simulink model "AIN_3x_6VT"  (R2018b)
settings: Solver=ode23t  StartTime=0.0  StopTime=0.3  RelTol=1e-3
undefined symbols (not defined in the file): C, DiscIntNeverNeededParam, fout, L, Rn
libraries: powerlib x38, powerlib_meascontrol x5, peRmsMeasurement x2, dspstat3 x1
settings Model: Creator=K2  LastModifiedBy=VID Company

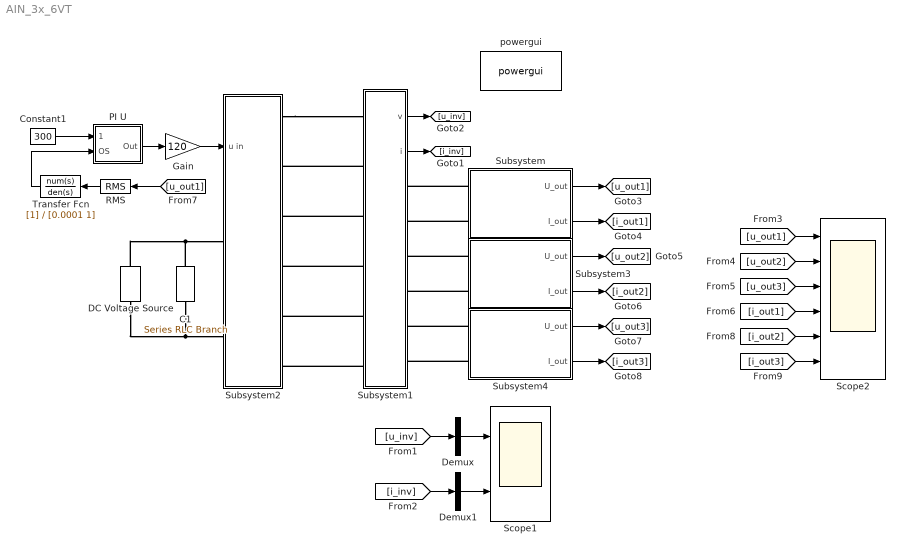
== system AIN_3x_6VT ==
  C1 : powerlib/Elements/Series RLC Branch  LConnTagsString=__new0  RConnTagsString=__new0  BranchType=RC  Resistance=0.050  Inductance=1e-3  SetiL0=off  InitialCurrent=0  Capacitance=10000e-6  Setx0=off  InitialVoltage=0  Measurements=None
  Constant1 : Constant  Value=300  SampleTime=1e-6
  DC Voltage Source : powerlib/Electrical Sources/DC Voltage Source  Amplitude=500  Measurements=None
  Demux : Demux  Outputs=3
  Demux1 : Demux  Outputs=3
  Gain : Gain  Gain=120
  PI U : Subsystem
  RMS : powerlib_meascontrol/Measurements/RMS  TrueRMS=off  Freq=400  RMSInit=0  Ts=0
  Scope1 : Scope  NumInputPorts=2
  Scope2 : Scope  NumInputPorts=6
  Subsystem : Subsystem
  Subsystem1 : Subsystem
  Subsystem2 : Subsystem
  Subsystem3 : Subsystem
  Subsystem4 : Subsystem
  Transfer Fcn : TransferFcn  Denominator=[0.0001 1]
  powergui : powerlib/powergui  Priority=1  SimulationMode=Discrete  SampleTime=1e-7  frequency=60  Iterations=50  frequencyindice=0  Pbase=100e6  ErrMax=1e-4  UnitsV=kV  UnitsW=MW  buscounter=0  FunctionMessages=off  echomessages=off  EnableUseOfTLC=off  CurrentSourceSwitches=off  DisableSnubberDevices=off  DisableRonSwitches=off  DisableVfSwitches=off  DisplayEquations=off  SolverType=Tustin/Backward Euler (TBE)  Interpol=off  ExternalGateDelay=off  methode=off  Ts=100  x0status=blocks  SPID=on  SwTol=0  HookPort=off  RestoreLinks=warning  ResistiveCurrentMeasurement=off  Frange=[0:2:500]  Ylog=off  Xlog=on  ShowGrid=off  save=off  variable=ZData  structure=logsout  ZoomFFT=on  StartTime=0.28  cycles=4  DisplayStyle=1  fundamental=400  FreqAxis=off  MaxFrequency=20000  frequencyindicesteady=1  RmsSteady=1  display=off
  wires:
  Constant1/1 -> PI U/1(Zad)
  RMS/1 -> Transfer Fcn/1
  Gain/1 -> Subsystem2/1(u in)
  PI U/1(Out) -> Gain/1
  Transfer Fcn/1 -> PI U/2(OS)
  Subsystem1/2(i) -> [i_inv]
  Subsystem1/1(v) -> [u_inv]
  [u_out1] -> RMS/1
  Subsystem/1(U_out) -> [u_out1]
  Subsystem/2(I_out) -> [i_out1]
  Subsystem3/1(U_out) -> [u_out2]
  Subsystem3/2(I_out) -> [i_out2]
  Subsystem4/1(U_out) -> [u_out3]
  Subsystem4/2(I_out) -> [i_out3]
  [u_out1] -> Scope2/1
  [u_out2] -> Scope2/2
  [u_out3] -> Scope2/3
  [i_out1] -> Scope2/4
  [i_out2] -> Scope2/5
  [i_out3] -> Scope2/6
  [u_inv] -> Demux/1
  [i_inv] -> Demux1/1
  Demux/2 -> Scope1/1
  Demux1/2 -> Scope1/2
  connections:
  DC Voltage Source/RConn1 -- C1/LConn1 -- Subsystem2/LConn1
  DC Voltage Source/LConn1 -- C1/RConn1 -- Subsystem2/LConn2
  Subsystem2/RConn1 -- Subsystem1/LConn1
  Subsystem1/LConn2 -- Subsystem2/RConn2
  Subsystem1/LConn4 -- Subsystem2/RConn4
  Subsystem1/LConn3 -- Subsystem2/RConn3
  Subsystem1/LConn5 -- Subsystem2/RConn5
  Subsystem1/LConn6 -- Subsystem2/RConn6
  Subsystem/LConn1 -- Subsystem1/RConn1
  Subsystem/LConn2 -- Subsystem1/RConn2
  Subsystem3/LConn1 -- Subsystem1/RConn3
  Subsystem3/LConn2 -- Subsystem1/RConn4
  Subsystem4/LConn1 -- Subsystem1/RConn5
  Subsystem4/LConn2 -- Subsystem1/RConn6

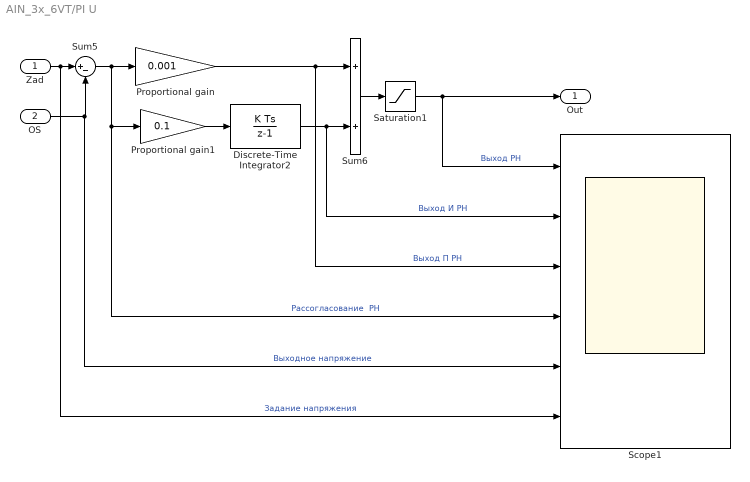
== system AIN_3x_6VT/PI U ==
  Zad : Inport
  OS : Inport  Port=2
  Discrete-Time Integrator2 : DiscreteIntegrator  SampleTime=-1  LimitOutput=on  UpperSaturationLimit=1  LowerSaturationLimit=0  ICPrevOutput=DiscIntNeverNeededParam  ICPrevScaledInput=DiscIntNeverNeededParam
  Proportional gain : Gain  Gain=0.001  SaturateOnIntegerOverflow=on  OutDataTypeStr=Inherit: Same as input  ParamDataTypeStr=Inherit: Same as input
  Proportional gain1 : Gain  Gain=0.1  SaturateOnIntegerOverflow=on  OutDataTypeStr=Inherit: Same as input  ParamDataTypeStr=Inherit: Same as input
  Saturation1 : Saturate  UpperLimit=1  LowerLimit=0
  Scope1 : Scope  NumInputPorts=6
  Sum5 : Sum  Inputs=|+-  SaturateOnIntegerOverflow=on  InputSameDT=on  OutDataTypeStr=Inherit: Same as first input
  Sum6 : Sum  SaturateOnIntegerOverflow=on  InputSameDT=on  OutDataTypeStr=Inherit: Same as first input
  Out : Outport
  wires:
  Proportional gain/1 -> Scope1/3, Sum6/1  "Выход П РН"
  Discrete-Time Integrator2/1 -> Sum6/2, Scope1/2  "Выход И РН"
  OS/1 -> Scope1/5, Sum5/2  "Выходное напряжение"
  Zad/1 -> Scope1/6, Sum5/1  "Задание напряжения"
  Sum5/1 -> Proportional gain1/1, Scope1/4, Proportional gain/1  "Рассогласование  РН"
  Sum6/1 -> Saturation1/1
  Saturation1/1 -> Out/1, Scope1/1  "Выход РН"
  Proportional gain1/1 -> Discrete-Time Integrator2/1

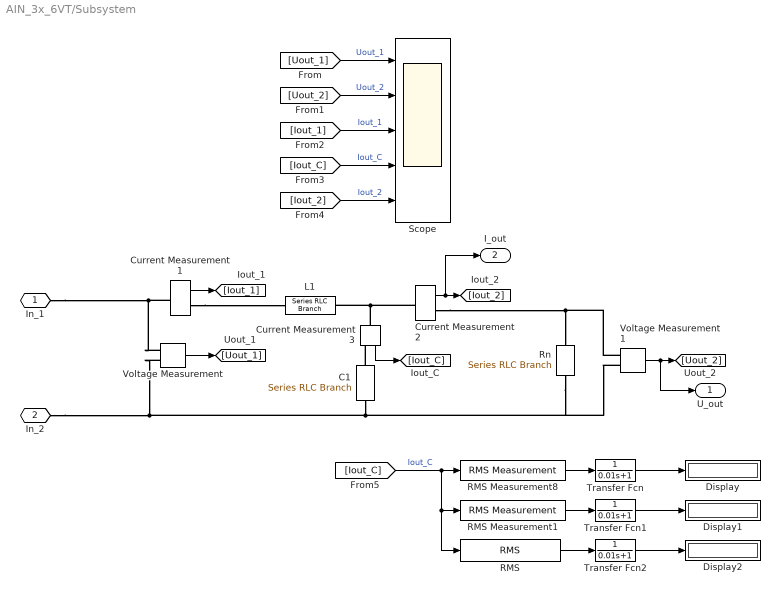
== system AIN_3x_6VT/Subsystem ==
  C1 : powerlib/Elements/Series RLC Branch  LConnTagsString=__new0  RConnTagsString=__new0  BranchType=RC  Resistance=0.050  Inductance=1e-3  SetiL0=off  InitialCurrent=0  Capacitance=C  Setx0=off  InitialVoltage=0  Measurements=None
  Current Measurement1 : powerlib/Measurements/Current Measurement  PhasorSimulation=off  OutputType=Complex  PSBequivalent=0
  Current Measurement2 : powerlib/Measurements/Current Measurement  PhasorSimulation=off  OutputType=Complex  PSBequivalent=0
  Current Measurement3 : powerlib/Measurements/Current Measurement  PhasorSimulation=off  OutputType=Complex  PSBequivalent=0
  Display : Display
  Display1 : Display
  Display2 : Display
  L1 : powerlib/Elements/Series RLC Branch  LConnTagsString=__new0  RConnTagsString=__new0  BranchType=RL  Resistance=0.1  Inductance=L  SetiL0=off  InitialCurrent=0  Capacitance=10e-3  Setx0=off  InitialVoltage=0  Measurements=None
  RMS : dspstat3/RMS  run=off  directionMode=Each column  dimension=1  InputProcessing=Columns as channels (frame based)  reset_popup=None
  RMS Measurement1 : peRmsMeasurement/RMS Measurement  LabelModeActiveChoice=Harmonic  F=8000  SpecifyHarmonics=on  K=[1]  Ts=0
  RMS Measurement8 : peRmsMeasurement/RMS Measurement  LabelModeActiveChoice=Harmonic  F=400  SpecifyHarmonics=on  K=[1]  Ts=0
  Rn : powerlib/Elements/Series RLC Branch  LConnTagsString=__new0  RConnTagsString=__new0  BranchType=RL  Resistance=Rn  Inductance=0.01e-3  SetiL0=off  InitialCurrent=0  Capacitance=50e-6  Setx0=off  InitialVoltage=0  Measurements=None
  Scope : Scope  NumInputPorts=5
  Transfer Fcn : TransferFcn  Denominator=[0.01 1]
  Transfer Fcn1 : TransferFcn  Denominator=[0.01 1]
  Transfer Fcn2 : TransferFcn  Denominator=[0.01 1]
  Voltage Measurement : powerlib/Measurements/Voltage Measurement  PhasorSimulation=off  OutputType=Complex  PSBequivalent=0
  Voltage Measurement1 : powerlib/Measurements/Voltage Measurement  PhasorSimulation=off  OutputType=Complex  PSBequivalent=0
  In_1 : PMIOPort  Side=Left
  In_2 : PMIOPort  Port=2  Side=Left
  U_out : Outport
  I_out : Outport  Port=2
  wires:
  Voltage Measurement1/1 -> U_out/1, [Uout_2]
  Current Measurement1/1 -> [Iout_1]
  Current Measurement2/1 -> I_out/1, [Iout_2]
  Voltage Measurement/1 -> [Uout_1]
  Current Measurement3/1 -> [Iout_C]
  [Iout_C] -> Scope/4  "Iout_C"
  [Uout_2] -> Scope/2  "Uout_2"
  [Iout_1] -> Scope/3  "Iout_1"
  [Iout_2] -> Scope/5  "Iout_2"
  [Uout_1] -> Scope/1  "Uout_1"
  [Iout_C] -> RMS/1, RMS Measurement1/1, RMS Measurement8/1  "Iout_C"
  RMS Measurement8/1 -> Transfer Fcn/1
  RMS Measurement1/1 -> Transfer Fcn1/1
  Transfer Fcn/1 -> Display/1
  Transfer Fcn1/1 -> Display1/1
  Transfer Fcn2/1 -> Display2/1
  RMS/1 -> Transfer Fcn2/1
  connections:
  Current Measurement3/LConn1 -- Current Measurement2/LConn1 -- L1/RConn1
  Current Measurement1/LConn1 -- In_1/RConn1 -- Voltage Measurement/LConn1
  Voltage Measurement/LConn2 -- In_2/RConn1 -- C1/RConn1 -- Rn/RConn1 -- Voltage Measurement1/LConn2
  Voltage Measurement1/LConn1 -- Current Measurement2/RConn1 -- Rn/LConn1
  Current Measurement1/RConn1 -- L1/LConn1
  C1/LConn1 -- Current Measurement3/RConn1

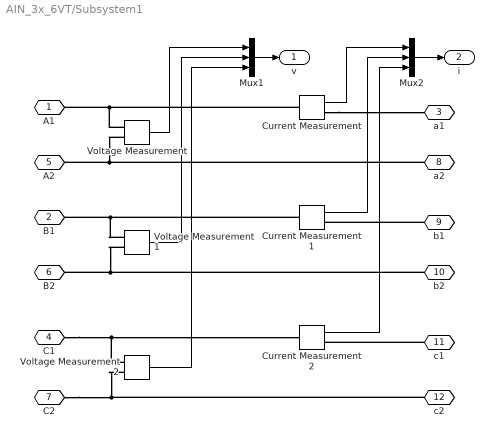
== system AIN_3x_6VT/Subsystem1 ==
  Current Measurement : powerlib/Measurements/Current Measurement  PhasorSimulation=off  OutputType=Complex  PSBequivalent=0
  Current Measurement1 : powerlib/Measurements/Current Measurement  PhasorSimulation=off  OutputType=Complex  PSBequivalent=0
  Current Measurement2 : powerlib/Measurements/Current Measurement  PhasorSimulation=off  OutputType=Complex  PSBequivalent=0
  Mux1 : Mux  Inputs=3
  Mux2 : Mux  Inputs=3
  Voltage Measurement : powerlib/Measurements/Voltage Measurement  PhasorSimulation=off  OutputType=Complex  PSBequivalent=0
  Voltage Measurement1 : powerlib/Measurements/Voltage Measurement  PhasorSimulation=off  OutputType=Complex  PSBequivalent=0
  Voltage Measurement2 : powerlib/Measurements/Voltage Measurement  PhasorSimulation=off  OutputType=Complex  PSBequivalent=0
  A1 : PMIOPort  Side=Left
  B1 : PMIOPort  Port=2  Side=Left
  a1 : PMIOPort  Port=3  Side=Right
  C1 : PMIOPort  Port=4  Side=Left
  A2 : PMIOPort  Port=5  Side=Left
  B2 : PMIOPort  Port=6  Side=Left
  C2 : PMIOPort  Port=7  Side=Left
  a2 : PMIOPort  Port=8  Side=Right
  b1 : PMIOPort  Port=9  Side=Right
  b2 : PMIOPort  Port=10  Side=Right
  c1 : PMIOPort  Port=11  Side=Right
  c2 : PMIOPort  Port=12  Side=Right
  v : Outport
  i : Outport  Port=2
  wires:
  Voltage Measurement1/1 -> Mux1/2
  Current Measurement2/1 -> Mux2/3
  Voltage Measurement2/1 -> Mux1/3
  Current Measurement/1 -> Mux2/1
  Voltage Measurement/1 -> Mux1/1
  Mux1/1 -> v/1
  Current Measurement1/1 -> Mux2/2
  Mux2/1 -> i/1
  connections:
  Current Measurement/RConn1 -- a1/RConn1
  Current Measurement/LConn1 -- Voltage Measurement/LConn1 -- A1/RConn1
  C1/RConn1 -- Voltage Measurement2/LConn1 -- Current Measurement2/LConn1
  c1/RConn1 -- Current Measurement2/RConn1
  Current Measurement1/LConn1 -- Voltage Measurement1/LConn1 -- B1/RConn1
  b1/RConn1 -- Current Measurement1/RConn1
  Voltage Measurement/LConn2 -- a2/RConn1 -- A2/RConn1
  Voltage Measurement1/LConn2 -- b2/RConn1 -- B2/RConn1
  Voltage Measurement2/LConn2 -- c2/RConn1 -- C2/RConn1

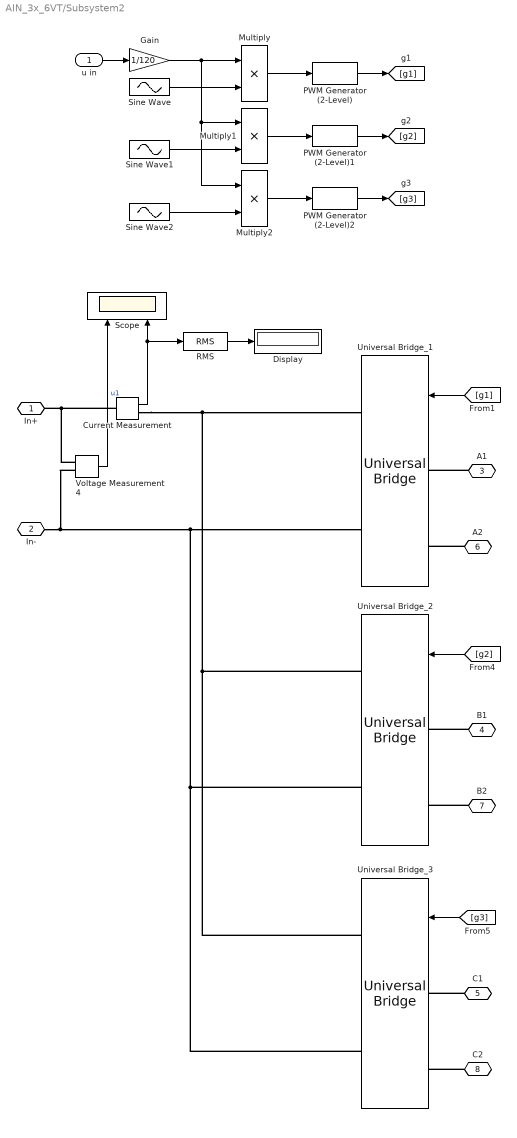
== system AIN_3x_6VT/Subsystem2 ==
  u in : Inport
  Current Measurement : powerlib/Measurements/Current Measurement  PhasorSimulation=off  OutputType=Complex  PSBequivalent=0
  Display : Display
  Gain : Gain  Gain=1/120
  Multiply : Product
  Multiply1 : Product
  Multiply2 : Product
  PWM Generator (2-Level) : powerlib_meascontrol/Pulse & Signal Generators/PWM Generator (2-Level)  ModulatorType=Single-phase full-bridge (4 pulses)  ModulatorMode=Unsynchronized  Fc=fPWM  Pc=0  nF=27  MinMax="[ -1  1 ]"  SamplingTechnique=Symmetrical regular (single edge)  ModulatingSignals=off  m=0.8  Freq=60  Phase=0  Ts=0  ShowCarrierOutport=off
      settings: SourceProductName=Simscape Power Systems
  PWM Generator (2-Level)1 : powerlib_meascontrol/Pulse & Signal Generators/PWM Generator (2-Level)  ModulatorType=Single-phase full-bridge (4 pulses)  ModulatorMode=Unsynchronized  Fc=fPWM  Pc=120  nF=27  MinMax="[ -1  1 ]"  SamplingTechnique=Symmetrical regular (single edge)  ModulatingSignals=off  m=0.8  Freq=60  Phase=0  Ts=0  ShowCarrierOutport=off
      settings: SourceProductName=Simscape Power Systems
  PWM Generator (2-Level)2 : powerlib_meascontrol/Pulse & Signal Generators/PWM Generator (2-Level)  ModulatorType=Single-phase full-bridge (4 pulses)  ModulatorMode=Unsynchronized  Fc=fPWM  Pc=240  nF=27  MinMax="[ -1  1 ]"  SamplingTechnique=Symmetrical regular (single edge)  ModulatingSignals=off  m=0.8  Freq=60  Phase=0  Ts=0  ShowCarrierOutport=off
      settings: SourceProductName=Simscape Power Systems
  RMS : powerlib_meascontrol/Measurements/RMS  TrueRMS=on  Freq=60  RMSInit=120  Ts=0
  Scope : Scope  NumInputPorts=2
  Sine Wave : Sin  Amplitude=0.99  Frequency=fout*2*pi  SampleTime=0
  Sine Wave1 : Sin  Amplitude=0.99  Frequency=fout*2*pi  Phase=2*pi*fout*(120/360)  SampleTime=0
  Sine Wave2 : Sin  Amplitude=0.99  Frequency=fout*2*pi  Phase=2*pi*fout*(240/360)  SampleTime=0
  Universal Bridge_1 : powerlib/Power Electronics/Universal Bridge  Arms=2  SnubberResistance=1e5  SnubberCapacitance=inf  Device=IGBT / Diodes  Ron=5e-3  Lon=0  ForwardVoltages="[  1.5  1  ]"  ForwardVoltage=0  GTOparameters=[ 10e-6 , 20e-6 ]  IGBTparameters=[ 1e-6 , 2e-6 ]  Measurements=Device currents  Measurements_2=None  converterType=Rectifier
  Universal Bridge_2 : powerlib/Power Electronics/Universal Bridge  Arms=2  SnubberResistance=1e5  SnubberCapacitance=inf  Device=IGBT / Diodes  Ron=5e-3  Lon=0  ForwardVoltages="[  1.5  1  ]"  ForwardVoltage=0  GTOparameters=[ 10e-6 , 20e-6 ]  IGBTparameters=[ 1e-6 , 2e-6 ]  Measurements=None  Measurements_2=None  converterType=Rectifier
  Universal Bridge_3 : powerlib/Power Electronics/Universal Bridge  Arms=2  SnubberResistance=1e5  SnubberCapacitance=inf  Device=IGBT / Diodes  Ron=5e-3  Lon=0  ForwardVoltages="[  1.5  1  ]"  ForwardVoltage=0  GTOparameters=[ 10e-6 , 20e-6 ]  IGBTparameters=[ 1e-6 , 2e-6 ]  Measurements=None  Measurements_2=None  converterType=Rectifier
  Voltage Measurement4 : powerlib/Measurements/Voltage Measurement  PhasorSimulation=off  OutputType=Complex  PSBequivalent=0
  In+ : PMIOPort  Side=Left
  In- : PMIOPort  Port=2  Side=Left
  A1 : PMIOPort  Port=3  Side=Right
  B1 : PMIOPort  Port=4  Side=Right
  C1 : PMIOPort  Port=5  Side=Right
  A2 : PMIOPort  Port=6  Side=Right
  B2 : PMIOPort  Port=7  Side=Right
  C2 : PMIOPort  Port=8  Side=Right
  wires:
  PWM Generator (2-Level)/1 -> [g1]
  Gain/1 -> Multiply2/1, Multiply1/1, Multiply/1
  u in/1 -> Gain/1
  Multiply/1 -> PWM Generator (2-Level)/1
  Sine Wave/1 -> Multiply/2
  Current Measurement/1 -> RMS/1, Scope/2
  Voltage Measurement4/1 -> Scope/1  "u1"
  Multiply1/1 -> PWM Generator (2-Level)1/1
  Multiply2/1 -> PWM Generator (2-Level)2/1
  PWM Generator (2-Level)2/1 -> [g3]
  PWM Generator (2-Level)1/1 -> [g2]
  [g1] -> Universal Bridge_1/1
  [g2] -> Universal Bridge_2/1
  [g3] -> Universal Bridge_3/1
  Sine Wave2/1 -> Multiply2/2
  Sine Wave1/1 -> Multiply1/2
  RMS/1 -> Display/1
  connections:
  Current Measurement/LConn1 -- Voltage Measurement4/LConn1 -- In+/RConn1
  In-/RConn1 -- Voltage Measurement4/LConn2 -- Universal Bridge_3/RConn2 -- Universal Bridge_2/RConn2 -- Universal Bridge_1/RConn2
  Current Measurement/RConn1 -- Universal Bridge_2/RConn1 -- Universal Bridge_3/RConn1 -- Universal Bridge_1/RConn1
  A1/RConn1 -- Universal Bridge_1/LConn1
  B1/RConn1 -- Universal Bridge_2/LConn1
  C1/RConn1 -- Universal Bridge_3/LConn1
  A2/RConn1 -- Universal Bridge_1/LConn2
  B2/RConn1 -- Universal Bridge_2/LConn2
  C2/RConn1 -- Universal Bridge_3/LConn2

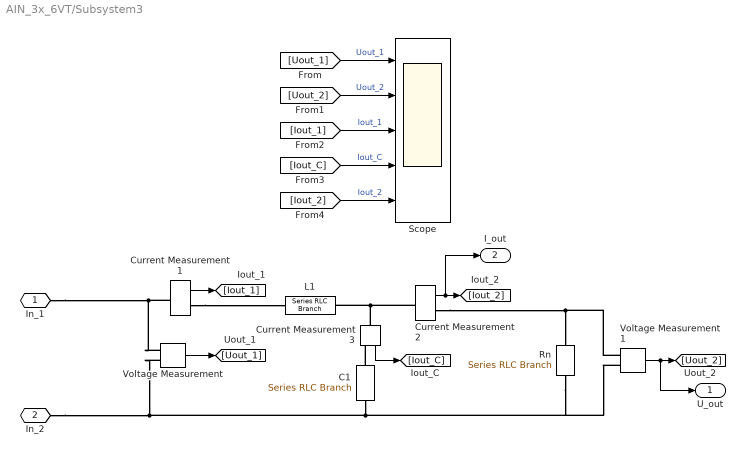
== system AIN_3x_6VT/Subsystem3 ==
  C1 : powerlib/Elements/Series RLC Branch  LConnTagsString=__new0  RConnTagsString=__new0  BranchType=RC  Resistance=0.050  Inductance=1e-3  SetiL0=off  InitialCurrent=0  Capacitance=C  Setx0=off  InitialVoltage=0  Measurements=None
  Current Measurement1 : powerlib/Measurements/Current Measurement  PhasorSimulation=off  OutputType=Complex  PSBequivalent=0
  Current Measurement2 : powerlib/Measurements/Current Measurement  PhasorSimulation=off  OutputType=Complex  PSBequivalent=0
  Current Measurement3 : powerlib/Measurements/Current Measurement  PhasorSimulation=off  OutputType=Complex  PSBequivalent=0
  L1 : powerlib/Elements/Series RLC Branch  LConnTagsString=__new0  RConnTagsString=__new0  BranchType=RL  Resistance=0.1  Inductance=L  SetiL0=off  InitialCurrent=0  Capacitance=10e-3  Setx0=off  InitialVoltage=0  Measurements=None
  Rn : powerlib/Elements/Series RLC Branch  LConnTagsString=__new0  RConnTagsString=__new0  BranchType=RL  Resistance=Rn  Inductance=0.01e-3  SetiL0=off  InitialCurrent=0  Capacitance=50e-6  Setx0=off  InitialVoltage=0  Measurements=None
  Scope : Scope  NumInputPorts=5
  Voltage Measurement : powerlib/Measurements/Voltage Measurement  PhasorSimulation=off  OutputType=Complex  PSBequivalent=0
  Voltage Measurement1 : powerlib/Measurements/Voltage Measurement  PhasorSimulation=off  OutputType=Complex  PSBequivalent=0
  In_1 : PMIOPort  Side=Left
  In_2 : PMIOPort  Port=2  Side=Left
  U_out : Outport
  I_out : Outport  Port=2
  wires:
  Voltage Measurement1/1 -> U_out/1, [Uout_2]
  Current Measurement1/1 -> [Iout_1]
  Current Measurement2/1 -> I_out/1, [Iout_2]
  Voltage Measurement/1 -> [Uout_1]
  Current Measurement3/1 -> [Iout_C]
  [Iout_C] -> Scope/4  "Iout_C"
  [Uout_2] -> Scope/2  "Uout_2"
  [Iout_1] -> Scope/3  "Iout_1"
  [Iout_2] -> Scope/5  "Iout_2"
  [Uout_1] -> Scope/1  "Uout_1"
  connections:
  Current Measurement3/LConn1 -- Current Measurement2/LConn1 -- L1/RConn1
  Current Measurement1/LConn1 -- In_1/RConn1 -- Voltage Measurement/LConn1
  Voltage Measurement/LConn2 -- In_2/RConn1 -- C1/RConn1 -- Rn/RConn1 -- Voltage Measurement1/LConn2
  Voltage Measurement1/LConn1 -- Current Measurement2/RConn1 -- Rn/LConn1
  Current Measurement1/RConn1 -- L1/LConn1
  C1/LConn1 -- Current Measurement3/RConn1

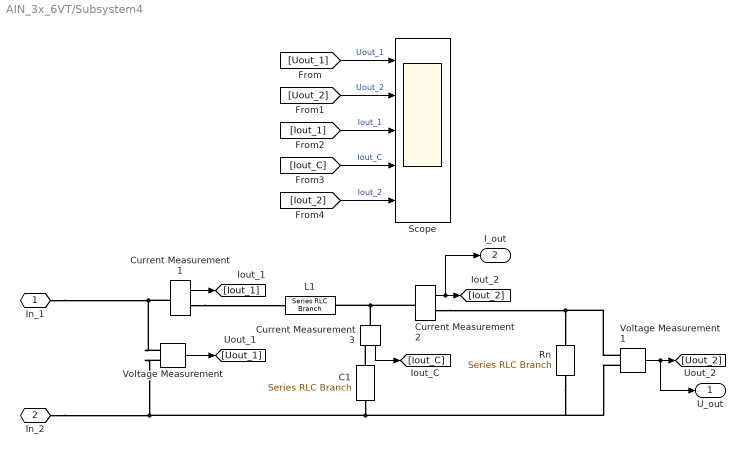
== system AIN_3x_6VT/Subsystem4 ==
  C1 : powerlib/Elements/Series RLC Branch  LConnTagsString=__new0  RConnTagsString=__new0  BranchType=RC  Resistance=0.050  Inductance=1e-3  SetiL0=off  InitialCurrent=0  Capacitance=C  Setx0=off  InitialVoltage=0  Measurements=None
  Current Measurement1 : powerlib/Measurements/Current Measurement  PhasorSimulation=off  OutputType=Complex  PSBequivalent=0
  Current Measurement2 : powerlib/Measurements/Current Measurement  PhasorSimulation=off  OutputType=Complex  PSBequivalent=0
  Current Measurement3 : powerlib/Measurements/Current Measurement  PhasorSimulation=off  OutputType=Complex  PSBequivalent=0
  L1 : powerlib/Elements/Series RLC Branch  LConnTagsString=__new0  RConnTagsString=__new0  BranchType=RL  Resistance=0.1  Inductance=L  SetiL0=off  InitialCurrent=0  Capacitance=10e-3  Setx0=off  InitialVoltage=0  Measurements=None
  Rn : powerlib/Elements/Series RLC Branch  LConnTagsString=__new0  RConnTagsString=__new0  BranchType=RL  Resistance=Rn  Inductance=0.01e-3  SetiL0=off  InitialCurrent=0  Capacitance=50e-6  Setx0=off  InitialVoltage=0  Measurements=None
  Scope : Scope  NumInputPorts=5
  Voltage Measurement : powerlib/Measurements/Voltage Measurement  PhasorSimulation=off  OutputType=Complex  PSBequivalent=0
  Voltage Measurement1 : powerlib/Measurements/Voltage Measurement  PhasorSimulation=off  OutputType=Complex  PSBequivalent=0
  In_1 : PMIOPort  Side=Left
  In_2 : PMIOPort  Port=2  Side=Left
  U_out : Outport
  I_out : Outport  Port=2
  wires:
  Voltage Measurement1/1 -> U_out/1, [Uout_2]
  Current Measurement1/1 -> [Iout_1]
  Current Measurement2/1 -> I_out/1, [Iout_2]
  Voltage Measurement/1 -> [Uout_1]
  Current Measurement3/1 -> [Iout_C]
  [Iout_C] -> Scope/4  "Iout_C"
  [Uout_2] -> Scope/2  "Uout_2"
  [Iout_1] -> Scope/3  "Iout_1"
  [Iout_2] -> Scope/5  "Iout_2"
  [Uout_1] -> Scope/1  "Uout_1"
  connections:
  Current Measurement3/LConn1 -- Current Measurement2/LConn1 -- L1/RConn1
  Current Measurement1/LConn1 -- In_1/RConn1 -- Voltage Measurement/LConn1
  Voltage Measurement/LConn2 -- In_2/RConn1 -- C1/RConn1 -- Rn/RConn1 -- Voltage Measurement1/LConn2
  Voltage Measurement1/LConn1 -- Current Measurement2/RConn1 -- Rn/LConn1
  Current Measurement1/RConn1 -- L1/LConn1
  C1/LConn1 -- Current Measurement3/RConn1
